simulink library "agg"  (Simulink 8.1)
settings: Solver=ode45  StartTime=0.0  StopTime=10.0  RelTol=1e-3
undefined symbols (not defined in the file or in its folder): C_TICK_TIME_S, FALSE, KIFO_AggressiveDriverTimer_ms, KIFO_SWSAggressiveDriver_degps, KIFO_ThrottlePosTimeDelay_ms, KIFO_ThrottleVariationAgg_pctps, TRUE
libraries: hcu_lib x2, idiada_lib x1
settings Model: Creator=xsellart  LastModifiedBy=tescamilla

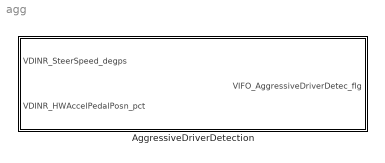
== system agg ==
  AggressiveDriverDetection : Subsystem

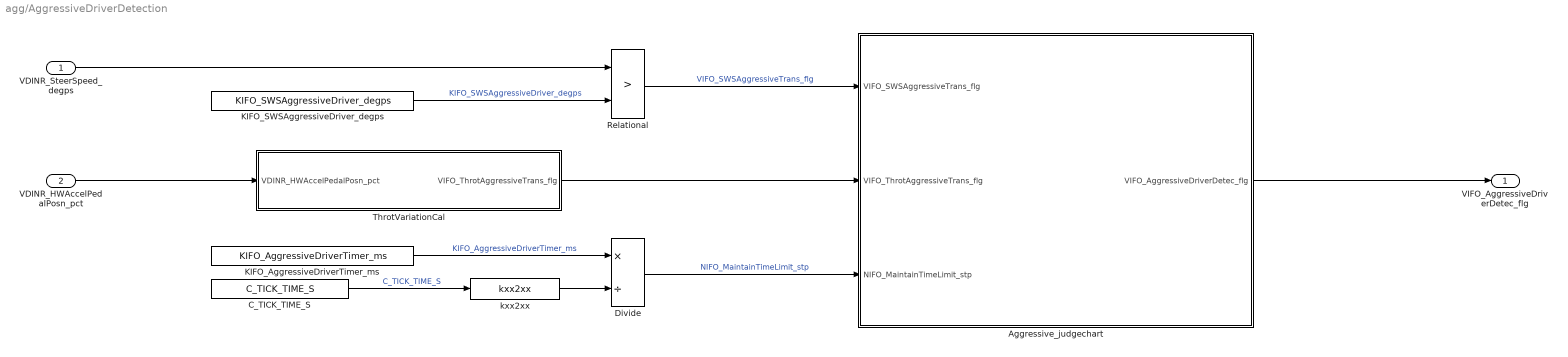
== system agg/AggressiveDriverDetection ==
  VDINR_SteerSpeed_degps : Inport
  VDINR_HWAccelPedalPosn_pct : Inport  Port=2
  Aggressive_judgechart : Stateflow chart  TreatAsAtomicUnit=on
  C_TICK_TIME_S : Constant  Value=C_TICK_TIME_S
  Divide : Product  Inputs=*/
  KIFO_AggressiveDriverTimer_ms : Constant  Value=KIFO_AggressiveDriverTimer_ms  OutDataTypeStr=single
  KIFO_SWSAggressiveDriver_degps : Constant  Value=KIFO_SWSAggressiveDriver_degps  OutDataTypeStr=single
  Relational : RelationalOperator  Operator=>  OutDataTypeStr=boolean
  ThrotVariationCal : Subsystem
  kxx2xx : hcu_lib/kxx2xx
  VIFO_AggressiveDriverDetec_flg : Outport
  wires:
  C_TICK_TIME_S/1 -> kxx2xx/1  "C_TICK_TIME_S"
  Divide/1 -> Aggressive_judgechart/3(NIFO_MaintainTimeLimit_stp)  "NIFO_MaintainTimeLimit_stp"
  kxx2xx/1 -> Divide/2
  KIFO_AggressiveDriverTimer_ms/1 -> Divide/1  "KIFO_AggressiveDriverTimer_ms"
  VDINR_SteerSpeed_degps/1 -> Relational/1
  KIFO_SWSAggressiveDriver_degps/1 -> Relational/2  "KIFO_SWSAggressiveDriver_degps"
  VDINR_HWAccelPedalPosn_pct/1 -> ThrotVariationCal/1(VDINR_HWAccelPedalPosn_pct)
  Relational/1 -> Aggressive_judgechart/1(VIFO_SWSAggressiveTrans_flg)  "VIFO_SWSAggressiveTrans_flg"
  ThrotVariationCal/1(VIFO_ThrotAggressiveTrans_flg) -> Aggressive_judgechart/2(VIFO_ThrotAggressiveTrans_flg)
  Aggressive_judgechart/1(VIFO_AggressiveDriverDetec_flg) -> VIFO_AggressiveDriverDetec_flg/1

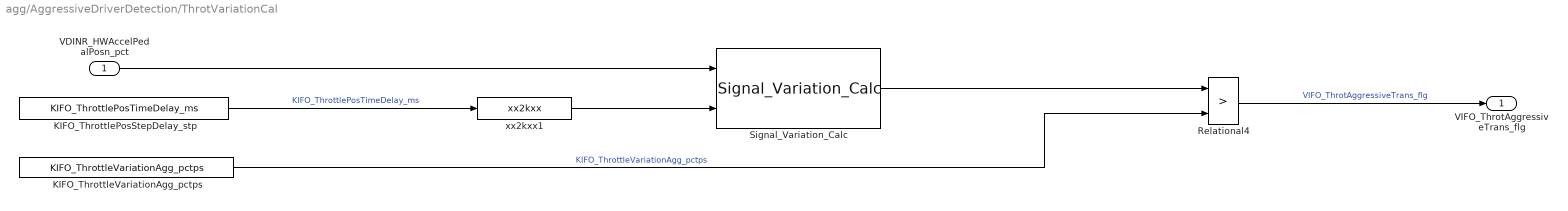
== system agg/AggressiveDriverDetection/ThrotVariationCal ==
  VDINR_HWAccelPedalPosn_pct : Inport
  KIFO_ThrottlePosStepDelay_stp : Constant  Value=KIFO_ThrottlePosTimeDelay_ms
  KIFO_ThrottleVariationAgg_pctps : Constant  Value=KIFO_ThrottleVariationAgg_pctps  OutDataTypeStr=single
  Relational4 : RelationalOperator  Operator=>  OutDataTypeStr=boolean
  Signal_Variation_Calc : idiada_lib/Signal_Variation_Calc
  xx2kxx1 : hcu_lib/xx2kxx
  VIFO_ThrotAggressiveTrans_flg : Outport
  wires:
  xx2kxx1/1 -> Signal_Variation_Calc/2
  VDINR_HWAccelPedalPosn_pct/1 -> Signal_Variation_Calc/1
  KIFO_ThrottlePosStepDelay_stp/1 -> xx2kxx1/1  "KIFO_ThrottlePosTimeDelay_ms"
  KIFO_ThrottleVariationAgg_pctps/1 -> Relational4/2  "KIFO_ThrottleVariationAgg_pctps"
  Signal_Variation_Calc/1 -> Relational4/1
  Relational4/1 -> VIFO_ThrotAggressiveTrans_flg/1  "VIFO_ThrotAggressiveTrans_flg"

== stateflow chart AggressiveDriverDetection/Aggressive_judgechart ==
  state OFF
    en:
    VIFO_AggressiveDriverDetec_flg = FALSE;
  state ON
    en:
    VIFO_AggressiveDriverDetec_flg = TRUE;
  state MAINTAIN
    en:
    NIFO_MaintainTimeLocal_stp = 0;
    du:
    NIFO_MaintainTimeLocal_stp = NIFO_MaintainTimeLocal_stp + 1;
  (default) -> OFF
  (junction 13) -> OFF : [NIFO_MaintainTimeLocal_stp > NIFO_MaintainTimeLimit_stp]
  MAINTAIN -> (junction 13) [order 2]
  OFF -> (junction 14)
  MAINTAIN -> ON [order 1] : [VIFO_SWSAggressiveTrans_flg==TRUE ...
      | || VIFO_ThrotAggressiveTrans_flg==TRUE]
  (junction 14) -> ON : [VIFO_SWSAggressiveTrans_flg==TRUE ...
      | || VIFO_ThrotAggressiveTrans_flg==TRUE]
  ON -> MAINTAIN : [VIFO_SWSAggressiveTrans_flg==FALSE ...
      | && VIFO_ThrotAggressiveTrans_flg==FALSE]
  data: VIFO_AggressiveDriverDetec_flg output boolean; VIFO_SWSAggressiveTrans_flg input boolean; VIFO_ThrotAggressiveTrans_flg input boolean; TRUE parameter double; FALSE parameter double; NIFO_MaintainTimeLocal_stp local single; NIFO_MaintainTimeLimit_stp input single
